simulink model "Project1"  (R2024a)
settings: Solver=VariableStepAuto  StartTime=0.0  StopTime=10.0  MaxStep=0.01  RelTol=1e-3
settings Model: Creator=harsh  LastModifiedBy=harsh

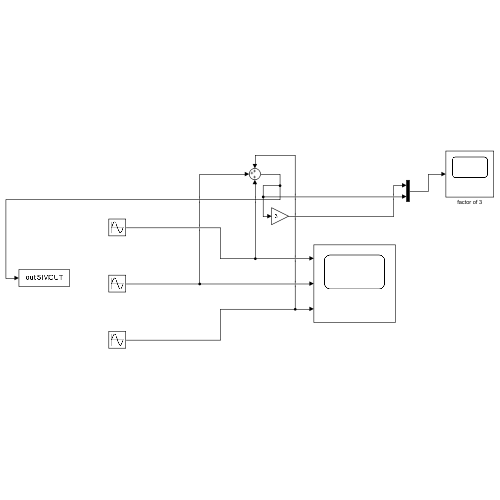
[thumbnail: Simulink's stored preview of the top-level diagram]
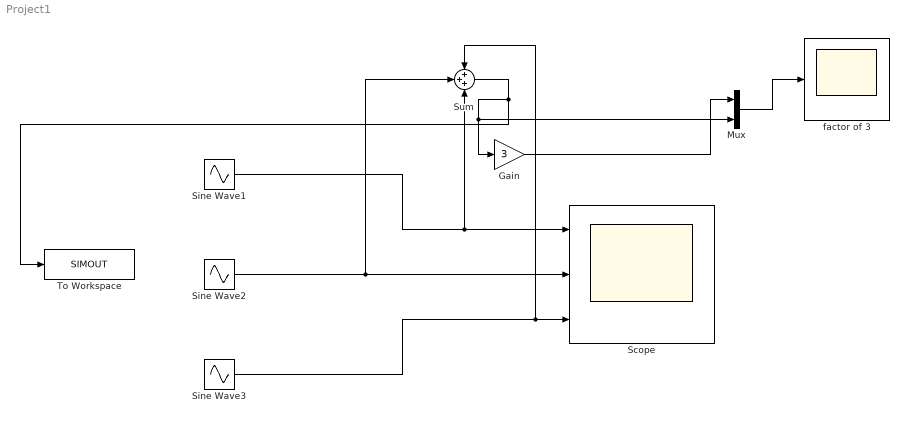
== system Project1 ==
  Gain : Gain  Gain=3
  Mux : Mux  Inputs=2
  Scope : Scope  NumInputPorts=3
  Sine Wave1 : Sin  SampleTime=0
  Sine Wave2 : Sin  Frequency=10  SampleTime=0
  Sine Wave3 : Sin  Frequency=20  SampleTime=0
  Sum : Sum  Inputs=+++
  To Workspace : ToWorkspace  VariableName=SIMOUT  SaveFormat=Timeseries  SampleTime=-1
  factor of 3 : Scope
  wires:
  Sine Wave1/1 -> Sum/3, Scope/1
  Sine Wave2/1 -> Sum/2, Scope/2
  Sine Wave3/1 -> Sum/1, Scope/3
  Sum/1 -> Gain/1, Mux/2, To Workspace/1
  Gain/1 -> Mux/1
  Mux/1 -> factor of 3/1
